simulink model "Controller"  (R2016b)
settings: Solver=ode45  StartTime=0.0  StopTime=330  MaxStep=0.01  RelTol=1e-3  EnableMultiTasking=on
values from neighbouring files (symbols this model uses):
  Controller_d_xc = 25.79    [Variables.m]
  Controller_d_yc = 0    [Variables.m]
  Controller_H = 115    [Variables.m]
  Controller_I_3 = 653.657    [Variables.m]
  Controller_I_L = 351.882    [Variables.m]
  Controller_I_p = 6428.68    [Variables.m]
  Controller_I_R = 351.882    [Variables.m]
  Controller_I_w3 = 628.378    [Variables.m]
  Controller_I_wL = 628.378    [Variables.m]
  Controller_I_wR = 628.378    [Variables.m]
  Controller_L = 107.8    [Variables.m]
  Controller_m_3 = 0.55    [Variables.m]
  Controller_m_L = 1.15    [Variables.m]
  Controller_m_p = 0.75    [Variables.m]
  Controller_m_R = 1.15    [Variables.m]
  Controller_R = 107.8    [Variables.m]
  Controller_R_3 = 50    [Variables.m]
  Controller_R_L = 50    [Variables.m]
  Controller_R_R = 50    [Variables.m]
  d_xc = 25    [Variables.m]
  d_yc = 0    [Variables.m]
  H = 115    [Variables.m]
  I_3 = 655    [Variables.m]
  I_L = 350    [Variables.m]
  I_p = 6430    [Variables.m]
  I_R = 350    [Variables.m]
  I_w3 = 629    [Variables.m]
  I_wL = 629    [Variables.m]
  I_wR = 629    [Variables.m]
  K_eta = diag([1, 1]) * 1.732    [Variables.m]
  K_eta_d = diag([1, 1]) * 0.5    [Variables.m]
  K_eta_i = diag([1, 1]) * 0.5    [Variables.m]
  K_theta = 0.016    [Variables.m]
  K_x = 10    [Variables.m]
  K_y = 0.000064    (= 6.4e-05)    [Variables.m]
  L = 108    [Variables.m]
  m_3 = 0.6    [Variables.m]
  m_L = 1.2    [Variables.m]
  m_p = 0.8    [Variables.m]
  m_R = 1.2    [Variables.m]
  maxTorque = 0    [Variables.m]
  R = 108    [Variables.m]
  R_3 = 52    [Variables.m]
  R_L = 49    [Variables.m]
  R_R = 51    [Variables.m]
undefined symbols (not defined in the file or in its folder): magnitude
settings Model: Creator=Vaibhav Gupta  LastModifiedBy=gupta
settings DataIOCC: ExternalInput=traj  LimitDataPoints=on  LoadExternalInput=on  SaveFormat=Array
settings OptimizationCC: LifeSpan=inf
settings DebuggingCC: SFUnexpectedBacktrackingDiag=warning  SFNoUnconditionalDefaultTransitionDiag=warning  SFExecutionAtInitializationDiag=none
settings HardwareCC: ProdBitPerPointer=32  ProdBitPerSizeT=32  ProdBitPerPtrDiffT=32  ProdLargestAtomicFloat=None  ProdIntDivRoundTo=Undefined  ProdEndianess=Unspecified  ProdWordSize=32  ProdHWDeviceType=32-bit Generic
settings ModelReferenceCC: PropagateSignalLabelsOutOfModel=off
settings GRTTargetCC: TargetLangStandard=C89/C90 (ANSI)  GeneratePreprocessorConditionals=Disable all
settings ConfigComp: CovMetricSettings=dw  CovHtmlReporting=on  CovSaveCumulativeToWorkspaceVar=on  CovSaveSingleToWorkspaceVar=on  CovExternalEMLEnable=off
settings ConfigurationSet: Description=SimMechanics 2G

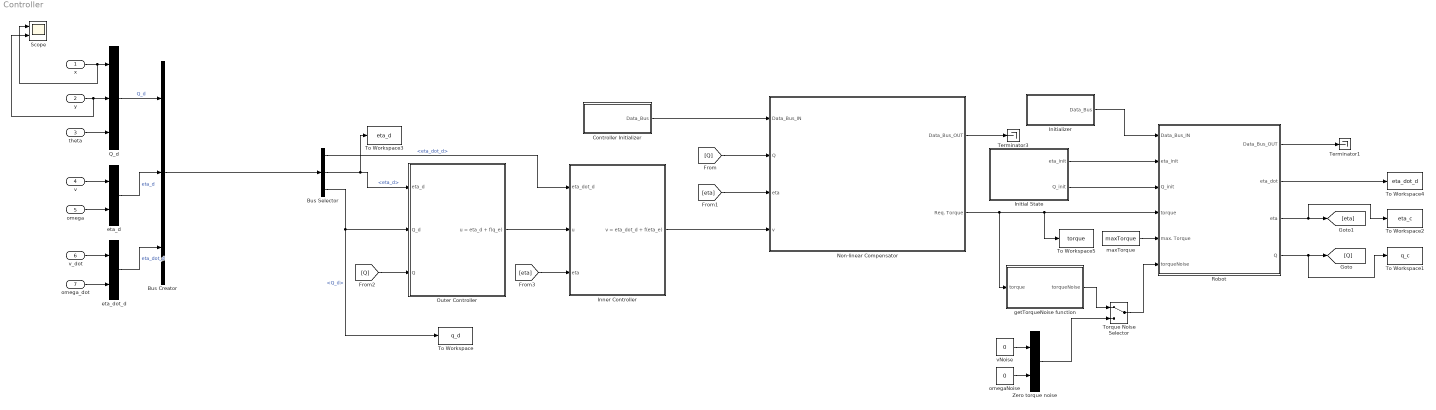
== system Controller ==
  x : Inport
  y : Inport  Port=2
  theta : Inport  Port=3
  v : Inport  Port=4
  omega : Inport  Port=5
  v_dot : Inport  Port=6
  omega_dot : Inport  Port=7
  Bus Creator : BusCreator  Inputs=3
  Bus Selector : BusSelector  OutputSignals=eta_dot_d,eta_d,Q_d
  Controller Initializer : Subsystem
  Initial State : Subsystem
  Initializer : Subsystem
  Inner Controller : Subsystem
  Non-linear Compensator : Subsystem
  Outer Controller : Subsystem
  Q_d : Concatenate  NumInputs=3
  Robot : Subsystem
  Scope : Scope  NumInputPorts=2
  Terminator1 : Terminator
  Terminator3 : Terminator
  To Workspace : ToWorkspace  VariableName=q_d  SaveFormat=Structure With Time  SampleTime=-1
      settings: Decimation=2
  To Workspace1 : ToWorkspace  VariableName=q_c  SaveFormat=Structure With Time  SampleTime=-1
      settings: Decimation=2
  To Workspace2 : ToWorkspace  VariableName=eta_c  SaveFormat=Structure With Time  SampleTime=-1
      settings: Decimation=2
  To Workspace3 : ToWorkspace  VariableName=eta_d  SaveFormat=Structure With Time  SampleTime=-1
      settings: Decimation=2
  To Workspace4 : ToWorkspace  VariableName=eta_dot_d  SaveFormat=Structure With Time  SampleTime=-1
      settings: Decimation=2
  To Workspace5 : ToWorkspace  VariableName=torque  SaveFormat=Structure With Time  SampleTime=-1
      settings: Decimation=2
  Torque Noise Selector : ManualSwitch
  Zero torque noise : Concatenate
  eta_d : Concatenate
  eta_dot_d : Concatenate
  getTorqueNoise function : MATLAB Function  TreatAsAtomicUnit=on
  maxTorque : Constant  Value=maxTorque
  omegaNoise : Constant  Value=0
  vNoise : Constant  Value=0
  wires:
  Robot/4(Q) -> To Workspace1/1, [Q]
  Robot/3(eta) -> [eta], To Workspace2/1
  Robot/1(Data_Bus_OUT) -> Terminator1/1
  Non-linear Compensator/2(Req. Torque) -> getTorqueNoise function/1(torque), To Workspace5/1, Robot/4(torque)
  [eta] -> Inner Controller/3(eta)
  [Q] -> Outer Controller/3(Q)
  Outer Controller/1(u = eta_d + f(q_e)) -> Inner Controller/2(u)
  Controller Initializer/1(Data_Bus) -> Non-linear Compensator/1(Data_Bus_IN)
  [eta] -> Non-linear Compensator/3(eta)
  [Q] -> Non-linear Compensator/2(Q)
  Inner Controller/1(v = eta_dot_d + f(eta_e)) -> Non-linear Compensator/4(v)
  Bus Selector/1 -> Inner Controller/1(eta_dot_d)  "<eta_dot_d>"
  Bus Selector/3 -> To Workspace/1, Outer Controller/2(Q_d)  "<Q_d>"
  Bus Selector/2 -> To Workspace3/1, Outer Controller/1(eta_d)  "<eta_d>"
  Initial State/1(eta_init) -> Robot/2(eta_init)
  Initial State/2(Q_init) -> Robot/3(Q_init)
  Bus Creator/1 -> Bus Selector/1
  Robot/2(eta_dot) -> To Workspace4/1
  v_dot/1 -> eta_dot_d/1
  omega/1 -> eta_d/2
  omega_dot/1 -> eta_dot_d/2
  theta/1 -> Q_d/3
  eta_dot_d/1 -> Bus Creator/3  "eta_dot_d"
  Q_d/1 -> Bus Creator/1  "Q_d"
  v/1 -> eta_d/1
  eta_d/1 -> Bus Creator/2  "eta_d"
  y/1 -> Scope/2, Q_d/2
  x/1 -> Scope/1, Q_d/1
  maxTorque/1 -> Robot/5(max. Torque)
  Initializer/1(Data_Bus) -> Robot/1(Data_Bus_IN)
  Non-linear Compensator/1(Data_Bus_OUT) -> Terminator3/1
  Torque Noise Selector/1 -> Robot/6(torqueNoise)
  getTorqueNoise function/1(torqueNoise) -> Torque Noise Selector/1
  omegaNoise/1 -> Zero torque noise/2
  vNoise/1 -> Zero torque noise/1
  Zero torque noise/1 -> Torque Noise Selector/2

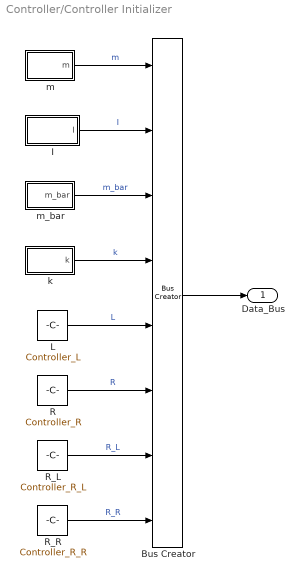
== system Controller/Controller Initializer ==
  Bus Creator : BusCreator  Inputs=8
  I : Subsystem
  L : Constant  Value=Controller_L
  R : Constant  Value=Controller_R
  R_L : Constant  Value=Controller_R_L
  R_R : Constant  Value=Controller_R_R
  k : Subsystem
  m : Subsystem
  m_bar : Subsystem
  Data_Bus : Outport
  wires:
  R_R/1 -> Bus Creator/8  "R_R"
  R_L/1 -> Bus Creator/7  "R_L"
  L/1 -> Bus Creator/5  "L"
  R/1 -> Bus Creator/6  "R"
  k/1(k) -> Bus Creator/4  "k"
  m/1(m) -> Bus Creator/1  "m"
  Bus Creator/1 -> Data_Bus/1
  m_bar/1(m_bar) -> Bus Creator/3  "m_bar"
  I/1(I) -> Bus Creator/2  "I"

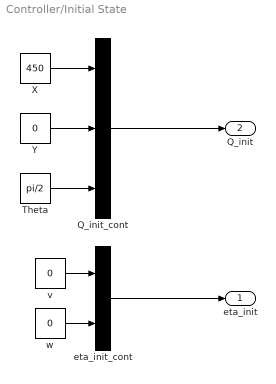
== system Controller/Initial State ==
  Q_init_cont : Concatenate  NumInputs=3
  Theta : Constant  Value=pi/2
  X : Constant  Value=450
  Y : Constant  Value=0
  eta_init_cont : Concatenate
  v : Constant  Value=0
  w : Constant  Value=0
  eta_init : Outport
  Q_init : Outport  Port=2
  wires:
  w/1 -> eta_init_cont/2
  Y/1 -> Q_init_cont/2
  Theta/1 -> Q_init_cont/3
  v/1 -> eta_init_cont/1
  X/1 -> Q_init_cont/1
  Q_init_cont/1 -> Q_init/1
  eta_init_cont/1 -> eta_init/1

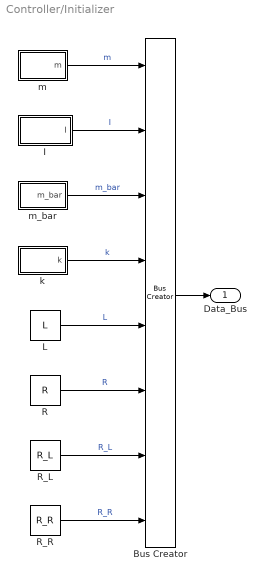
== system Controller/Initializer ==
  Bus Creator : BusCreator  Inputs=8
  I : Subsystem
  L : Constant  Value=L
  R : Constant  Value=R
  R_L : Constant  Value=R_L
  R_R : Constant  Value=R_R
  k : Subsystem
  m : Subsystem
  m_bar : Subsystem
  Data_Bus : Outport
  wires:
  I/1(I) -> Bus Creator/2  "I"
  m_bar/1(m_bar) -> Bus Creator/3  "m_bar"
  Bus Creator/1 -> Data_Bus/1
  m/1(m) -> Bus Creator/1  "m"
  k/1(k) -> Bus Creator/4  "k"
  R/1 -> Bus Creator/6  "R"
  L/1 -> Bus Creator/5  "L"
  R_L/1 -> Bus Creator/7  "R_L"
  R_R/1 -> Bus Creator/8  "R_R"

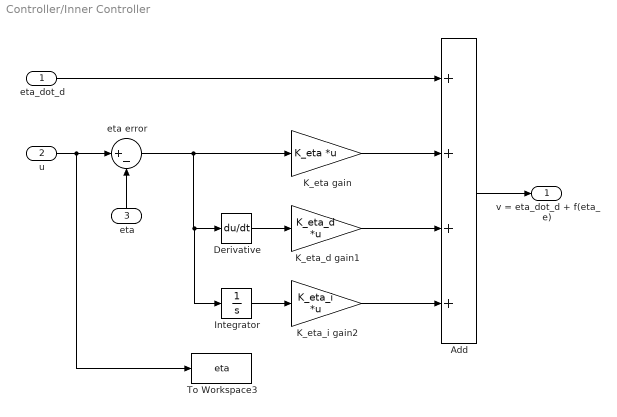
== system Controller/Inner Controller ==
  eta_dot_d : Inport
  u : Inport  Port=2
  eta : Inport  Port=3
  Add : Sum  Inputs=++++
  Derivative : Derivative  CoefficientInTFapproximation=100
  Integrator : Integrator  LimitOutput=on  UpperSaturationLimit=100  LowerSaturationLimit=-100
  K_eta gain : Gain  Gain=K_eta  Multiplication=Matrix(K*u) (u vector)
  K_eta_d gain1 : Gain  Gain=K_eta_d  Multiplication=Matrix(K*u) (u vector)
  K_eta_i gain2 : Gain  Gain=K_eta_i  Multiplication=Matrix(K*u) (u vector)
  To Workspace3 : ToWorkspace  VariableName=eta  SaveFormat=Structure With Time  SampleTime=-1
      settings: Decimation=2
  eta error : Sum  Inputs=|+-
  v = eta_dot_d + f(eta_e) : Outport
  wires:
  Add/1 -> v = eta_dot_d + f(eta_e)/1
  eta_dot_d/1 -> Add/1
  K_eta gain/1 -> Add/2
  eta error/1 -> Integrator/1, Derivative/1, K_eta gain/1
  u/1 -> To Workspace3/1, eta error/1
  eta/1 -> eta error/2
  K_eta_d gain1/1 -> Add/3
  Derivative/1 -> K_eta_d gain1/1
  Integrator/1 -> K_eta_i gain2/1
  K_eta_i gain2/1 -> Add/4

== system Controller/Non-linear Compensator ==
  Data_Bus_IN : Inport
  Q : Inport  Port=2
  eta : Inport  Port=3
  v : Inport  Port=4
  Bus Selector1 : BusSelector  OutputSignals=m,I,m_bar,k,L,R,R_L,R_R
  getTorque function : MATLAB Function  TreatAsAtomicUnit=on
  Data_Bus_OUT : Outport
  Req. Torque : Outport  Port=2
  wires:
  getTorque function/1(torque) -> Req. Torque/1
  Data_Bus_IN/1 -> Bus Selector1/1, Data_Bus_OUT/1
  v/1 -> getTorque function/11(v)
  eta/1 -> getTorque function/10(eta)
  Q/1 -> getTorque function/9(Q)
  Bus Selector1/1 -> getTorque function/1(M)  "<m>"
  Bus Selector1/2 -> getTorque function/2(I)  "<I>"
  Bus Selector1/3 -> getTorque function/3(M_bar)  "<m_bar>"
  Bus Selector1/4 -> getTorque function/4(k)  "<k>"
  Bus Selector1/5 -> getTorque function/5(L)  "<L>"
  Bus Selector1/6 -> getTorque function/6(R)  "<R>"
  Bus Selector1/7 -> getTorque function/7(R_L)  "<R_L>"
  Bus Selector1/8 -> getTorque function/8(R_R)  "<R_R>"

== system Controller/Outer Controller ==
  eta_d : Inport
  Q_d : Inport  Port=2
  Q : Inport  Port=3
  K_theta : Constant  Value=K_theta
  K_x : Constant  Value=K_x
  K_y : Constant  Value=K_y
  Q error : Sum  Inputs=|+-
  getX function : MATLAB Function  TreatAsAtomicUnit=on
  u = eta_d + f(q_e) : Outport
  wires:
  Q_d/1 -> Q error/1
  Q/1 -> getX function/6(Q), Q error/2
  Q error/1 -> getX function/5(Q_e)
  eta_d/1 -> getX function/1(eta_d)
  getX function/1(x) -> u = eta_d + f(q_e)/1
  K_x/1 -> getX function/2(K_x)
  K_y/1 -> getX function/3(K_y)
  K_theta/1 -> getX function/4(K_theta)

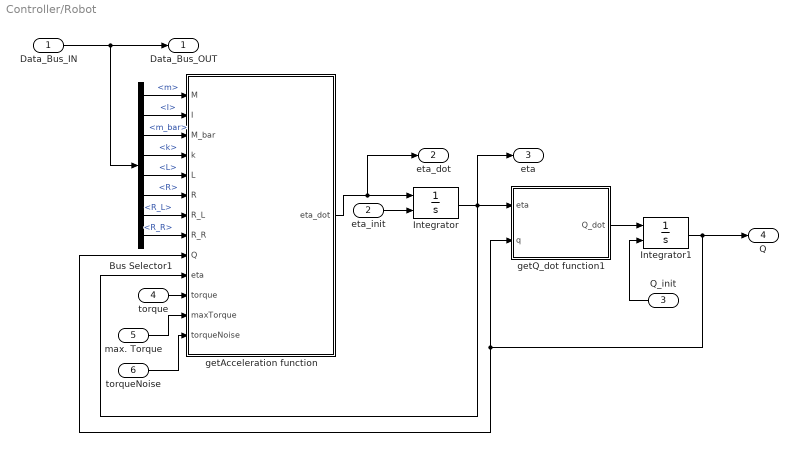
== system Controller/Robot ==
  Data_Bus_IN : Inport
  eta_init : Inport  Port=2
  Q_init : Inport  Port=3
  torque : Inport  Port=4
  max. Torque : Inport  Port=5
  torqueNoise : Inport  Port=6
  Bus Selector1 : BusSelector  OutputSignals=m,I,m_bar,k,L,R,R_L,R_R
  Integrator : Integrator  InitialConditionSource=external  UpperSaturationLimit=10  LowerSaturationLimit=-10
  Integrator1 : Integrator  InitialConditionSource=external
  getAcceleration function : MATLAB Function  TreatAsAtomicUnit=on
  getQ_dot function1 : MATLAB Function  TreatAsAtomicUnit=on
  Data_Bus_OUT : Outport
  eta_dot : Outport  Port=2
  eta : Outport  Port=3
  Q : Outport  Port=4
  wires:
  Integrator/1 -> getQ_dot function1/1(eta), getAcceleration function/10(eta), eta/1
  Integrator1/1 -> getQ_dot function1/2(q), getAcceleration function/9(Q), Q/1
  Bus Selector1/1 -> getAcceleration function/1(M)  "<m>"
  Q_init/1 -> Integrator1/2
  eta_init/1 -> Integrator/2
  torque/1 -> getAcceleration function/11(torque)
  Bus Selector1/2 -> getAcceleration function/2(I)  "<I>"
  Data_Bus_IN/1 -> Bus Selector1/1, Data_Bus_OUT/1
  getAcceleration function/1(eta_dot) -> Integrator/1, eta_dot/1
  Bus Selector1/3 -> getAcceleration function/3(M_bar)  "<m_bar>"
  Bus Selector1/4 -> getAcceleration function/4(k)  "<k>"
  Bus Selector1/5 -> getAcceleration function/5(L)  "<L>"
  Bus Selector1/6 -> getAcceleration function/6(R)  "<R>"
  Bus Selector1/7 -> getAcceleration function/7(R_L)  "<R_L>"
  Bus Selector1/8 -> getAcceleration function/8(R_R)  "<R_R>"
  getQ_dot function1/1(Q_dot) -> Integrator1/1
  max. Torque/1 -> getAcceleration function/12(maxTorque)
  torqueNoise/1 -> getAcceleration function/13(torqueNoise)

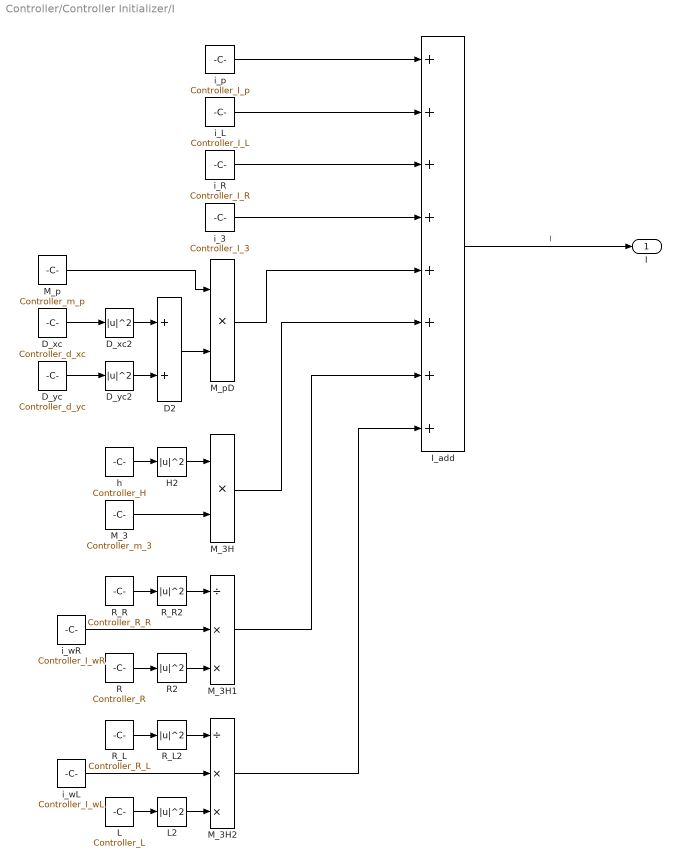
== system Controller/Controller Initializer/I ==
  D2 : Sum
  D_xc : Constant  Value=Controller_d_xc
  D_xc2 : Math  Operator=magnitude^2  SaturateOnIntegerOverflow=on
  D_yc : Constant  Value=Controller_d_yc
  D_yc2 : Math  Operator=magnitude^2  SaturateOnIntegerOverflow=on
  H2 : Math  Operator=magnitude^2  SaturateOnIntegerOverflow=on
  I_add : Sum  Inputs=++++++++
  L : Constant  Value=Controller_L
  L2 : Math  Operator=magnitude^2  SaturateOnIntegerOverflow=on
  M_3 : Constant  Value=Controller_m_3
  M_3H : Product  Inputs=**
  M_3H1 : Product  Inputs=/**
  M_3H2 : Product  Inputs=/**
  M_p : Constant  Value=Controller_m_p
  M_pD : Product  Inputs=**
  R : Constant  Value=Controller_R
  R2 : Math  Operator=magnitude^2  SaturateOnIntegerOverflow=on
  R_L : Constant  Value=Controller_R_L
  R_L2 : Math  Operator=magnitude^2  SaturateOnIntegerOverflow=on
  R_R : Constant  Value=Controller_R_R
  R_R2 : Math  Operator=magnitude^2  SaturateOnIntegerOverflow=on
  h : Constant  Value=Controller_H
  i_3 : Constant  Value=Controller_I_3
  i_L : Constant  Value=Controller_I_L
  i_R : Constant  Value=Controller_I_R
  i_p : Constant  Value=Controller_I_p
  i_wL : Constant  Value=Controller_I_wL
  i_wR : Constant  Value=Controller_I_wR
  I : Outport
  wires:
  i_wL/1 -> M_3H2/2
  L2/1 -> M_3H2/3
  L/1 -> L2/1
  R_L2/1 -> M_3H2/1
  R_L/1 -> R_L2/1
  M_3H2/1 -> I_add/8
  i_wR/1 -> M_3H1/2
  R2/1 -> M_3H1/3
  R/1 -> R2/1
  R_R2/1 -> M_3H1/1
  R_R/1 -> R_R2/1
  M_3H1/1 -> I_add/7
  i_p/1 -> I_add/1
  i_L/1 -> I_add/2
  i_R/1 -> I_add/3
  i_3/1 -> I_add/4
  I_add/1 -> I/1  "I"
  M_p/1 -> M_pD/1
  D_xc/1 -> D_xc2/1
  D_yc/1 -> D_yc2/1
  D_xc2/1 -> D2/1
  D_yc2/1 -> D2/2
  D2/1 -> M_pD/2
  M_pD/1 -> I_add/5
  H2/1 -> M_3H/1
  h/1 -> H2/1
  M_3/1 -> M_3H/2
  M_3H/1 -> I_add/6

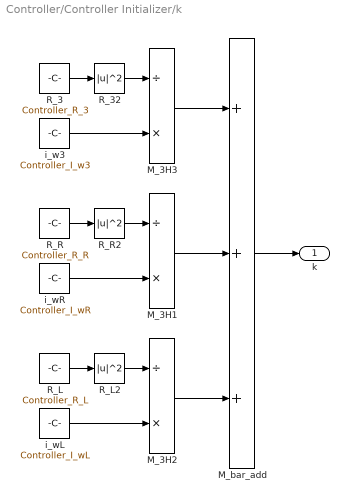
== system Controller/Controller Initializer/k ==
  M_3H1 : Product  Inputs=/*
  M_3H2 : Product  Inputs=/*
  M_3H3 : Product  Inputs=/*
  M_bar_add : Sum  Inputs=+++
  R_3 : Constant  Value=Controller_R_3
  R_32 : Math  Operator=magnitude^2  SaturateOnIntegerOverflow=on
  R_L : Constant  Value=Controller_R_L
  R_L2 : Math  Operator=magnitude^2  SaturateOnIntegerOverflow=on
  R_R : Constant  Value=Controller_R_R
  R_R2 : Math  Operator=magnitude^2  SaturateOnIntegerOverflow=on
  i_w3 : Constant  Value=Controller_I_w3
  i_wL : Constant  Value=Controller_I_wL
  i_wR : Constant  Value=Controller_I_wR
  k : Outport
  wires:
  M_3H3/1 -> M_bar_add/1
  i_w3/1 -> M_3H3/2
  R_32/1 -> M_3H3/1
  R_3/1 -> R_32/1
  M_3H1/1 -> M_bar_add/2
  M_3H2/1 -> M_bar_add/3
  i_wL/1 -> M_3H2/2
  R_L2/1 -> M_3H2/1
  R_L/1 -> R_L2/1
  i_wR/1 -> M_3H1/2
  R_R2/1 -> M_3H1/1
  R_R/1 -> R_R2/1
  M_bar_add/1 -> k/1

== system Controller/Controller Initializer/m ==
  M_3 : Constant  Value=Controller_m_3
  M_L : Constant  Value=Controller_m_L
  M_R : Constant  Value=Controller_m_R
  M_add : Sum  Inputs=++++
  M_p : Constant  Value=Controller_m_p
  m : Outport
  wires:
  M_3/1 -> M_add/4
  M_L/1 -> M_add/2
  M_p/1 -> M_add/1
  M_R/1 -> M_add/3
  M_add/1 -> m/1  "m"

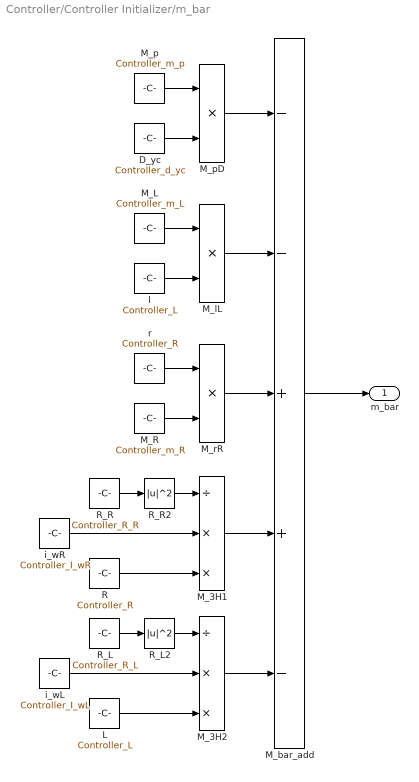
== system Controller/Controller Initializer/m_bar ==
  D_yc : Constant  Value=Controller_d_yc
  L : Constant  Value=Controller_L
  M_3H1 : Product  Inputs=/**
  M_3H2 : Product  Inputs=/**
  M_L : Constant  Value=Controller_m_L
  M_R : Constant  Value=Controller_m_R
  M_bar_add : Sum  Inputs=--++-
  M_lL : Product  Inputs=**
  M_p : Constant  Value=Controller_m_p
  M_pD : Product  Inputs=**
  M_rR : Product  Inputs=**
  R : Constant  Value=Controller_R
  R_L : Constant  Value=Controller_R_L
  R_L2 : Math  Operator=magnitude^2  SaturateOnIntegerOverflow=on
  R_R : Constant  Value=Controller_R_R
  R_R2 : Math  Operator=magnitude^2  SaturateOnIntegerOverflow=on
  i_wL : Constant  Value=Controller_I_wL
  i_wR : Constant  Value=Controller_I_wR
  l : Constant  Value=Controller_L
  r : Constant  Value=Controller_R
  m_bar : Outport
  wires:
  M_3H1/1 -> M_bar_add/4
  M_3H2/1 -> M_bar_add/5
  i_wL/1 -> M_3H2/2
  L/1 -> M_3H2/3
  R_L2/1 -> M_3H2/1
  R_L/1 -> R_L2/1
  i_wR/1 -> M_3H1/2
  R/1 -> M_3H1/3
  R_R2/1 -> M_3H1/1
  R_R/1 -> R_R2/1
  D_yc/1 -> M_pD/2
  M_p/1 -> M_pD/1
  l/1 -> M_lL/2
  M_L/1 -> M_lL/1
  M_R/1 -> M_rR/2
  r/1 -> M_rR/1
  M_pD/1 -> M_bar_add/1
  M_lL/1 -> M_bar_add/2
  M_rR/1 -> M_bar_add/3
  M_bar_add/1 -> m_bar/1

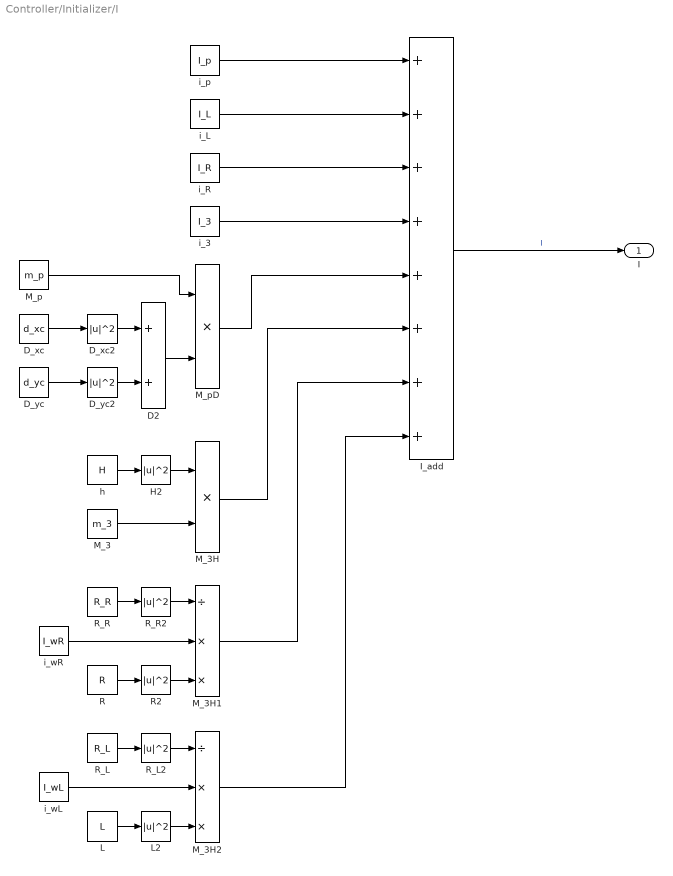
== system Controller/Initializer/I ==
  D2 : Sum
  D_xc : Constant  Value=d_xc
  D_xc2 : Math  Operator=magnitude^2  SaturateOnIntegerOverflow=on
  D_yc : Constant  Value=d_yc
  D_yc2 : Math  Operator=magnitude^2  SaturateOnIntegerOverflow=on
  H2 : Math  Operator=magnitude^2  SaturateOnIntegerOverflow=on
  I_add : Sum  Inputs=++++++++
  L : Constant  Value=L
  L2 : Math  Operator=magnitude^2  SaturateOnIntegerOverflow=on
  M_3 : Constant  Value=m_3
  M_3H : Product  Inputs=**
  M_3H1 : Product  Inputs=/**
  M_3H2 : Product  Inputs=/**
  M_p : Constant  Value=m_p
  M_pD : Product  Inputs=**
  R : Constant  Value=R
  R2 : Math  Operator=magnitude^2  SaturateOnIntegerOverflow=on
  R_L : Constant  Value=R_L
  R_L2 : Math  Operator=magnitude^2  SaturateOnIntegerOverflow=on
  R_R : Constant  Value=R_R
  R_R2 : Math  Operator=magnitude^2  SaturateOnIntegerOverflow=on
  h : Constant  Value=H
  i_3 : Constant  Value=I_3
  i_L : Constant  Value=I_L
  i_R : Constant  Value=I_R
  i_p : Constant  Value=I_p
  i_wL : Constant  Value=I_wL
  i_wR : Constant  Value=I_wR
  I : Outport
  wires:
  M_3H/1 -> I_add/6
  M_3/1 -> M_3H/2
  h/1 -> H2/1
  H2/1 -> M_3H/1
  M_pD/1 -> I_add/5
  D2/1 -> M_pD/2
  D_yc2/1 -> D2/2
  D_xc2/1 -> D2/1
  D_yc/1 -> D_yc2/1
  D_xc/1 -> D_xc2/1
  M_p/1 -> M_pD/1
  I_add/1 -> I/1  "I"
  i_3/1 -> I_add/4
  i_R/1 -> I_add/3
  i_L/1 -> I_add/2
  i_p/1 -> I_add/1
  M_3H1/1 -> I_add/7
  R_R/1 -> R_R2/1
  R_R2/1 -> M_3H1/1
  R/1 -> R2/1
  R2/1 -> M_3H1/3
  i_wR/1 -> M_3H1/2
  M_3H2/1 -> I_add/8
  R_L/1 -> R_L2/1
  R_L2/1 -> M_3H2/1
  L/1 -> L2/1
  L2/1 -> M_3H2/3
  i_wL/1 -> M_3H2/2

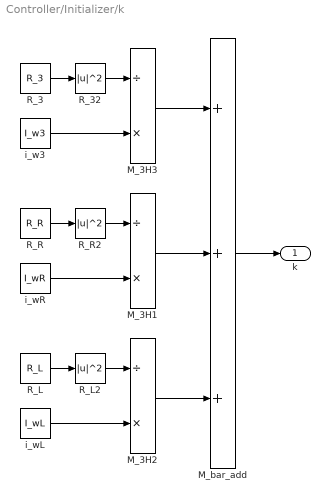
== system Controller/Initializer/k ==
  M_3H1 : Product  Inputs=/*
  M_3H2 : Product  Inputs=/*
  M_3H3 : Product  Inputs=/*
  M_bar_add : Sum  Inputs=+++
  R_3 : Constant  Value=R_3
  R_32 : Math  Operator=magnitude^2  SaturateOnIntegerOverflow=on
  R_L : Constant  Value=R_L
  R_L2 : Math  Operator=magnitude^2  SaturateOnIntegerOverflow=on
  R_R : Constant  Value=R_R
  R_R2 : Math  Operator=magnitude^2  SaturateOnIntegerOverflow=on
  i_w3 : Constant  Value=I_w3
  i_wL : Constant  Value=I_wL
  i_wR : Constant  Value=I_wR
  k : Outport
  wires:
  M_bar_add/1 -> k/1
  R_R/1 -> R_R2/1
  R_R2/1 -> M_3H1/1
  i_wR/1 -> M_3H1/2
  R_L/1 -> R_L2/1
  R_L2/1 -> M_3H2/1
  i_wL/1 -> M_3H2/2
  M_3H2/1 -> M_bar_add/3
  M_3H1/1 -> M_bar_add/2
  R_3/1 -> R_32/1
  R_32/1 -> M_3H3/1
  i_w3/1 -> M_3H3/2
  M_3H3/1 -> M_bar_add/1

== system Controller/Initializer/m ==
  M_3 : Constant  Value=m_3
  M_L : Constant  Value=m_L
  M_R : Constant  Value=m_R
  M_add : Sum  Inputs=++++
  M_p : Constant  Value=m_p
  m : Outport
  wires:
  M_add/1 -> m/1  "m"
  M_R/1 -> M_add/3
  M_p/1 -> M_add/1
  M_L/1 -> M_add/2
  M_3/1 -> M_add/4

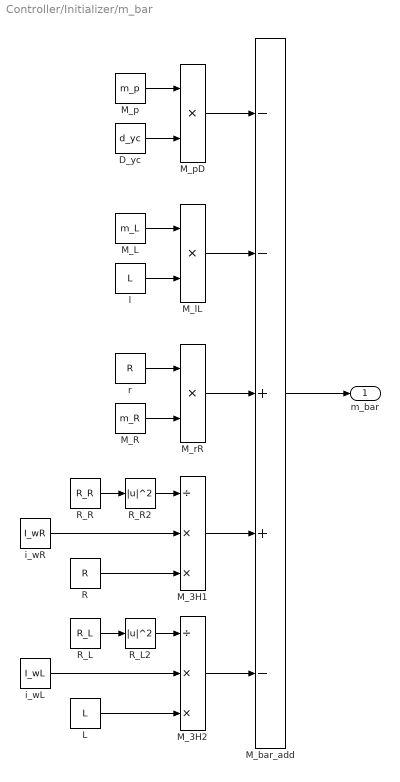
== system Controller/Initializer/m_bar ==
  D_yc : Constant  Value=d_yc
  L : Constant  Value=L
  M_3H1 : Product  Inputs=/**
  M_3H2 : Product  Inputs=/**
  M_L : Constant  Value=m_L
  M_R : Constant  Value=m_R
  M_bar_add : Sum  Inputs=--++-
  M_lL : Product  Inputs=**
  M_p : Constant  Value=m_p
  M_pD : Product  Inputs=**
  M_rR : Product  Inputs=**
  R : Constant  Value=R
  R_L : Constant  Value=R_L
  R_L2 : Math  Operator=magnitude^2  SaturateOnIntegerOverflow=on
  R_R : Constant  Value=R_R
  R_R2 : Math  Operator=magnitude^2  SaturateOnIntegerOverflow=on
  i_wL : Constant  Value=I_wL
  i_wR : Constant  Value=I_wR
  l : Constant  Value=L
  r : Constant  Value=R
  m_bar : Outport
  wires:
  M_bar_add/1 -> m_bar/1
  M_rR/1 -> M_bar_add/3
  M_lL/1 -> M_bar_add/2
  M_pD/1 -> M_bar_add/1
  r/1 -> M_rR/1
  M_R/1 -> M_rR/2
  M_L/1 -> M_lL/1
  l/1 -> M_lL/2
  M_p/1 -> M_pD/1
  D_yc/1 -> M_pD/2
  R_R/1 -> R_R2/1
  R_R2/1 -> M_3H1/1
  R/1 -> M_3H1/3
  i_wR/1 -> M_3H1/2
  R_L/1 -> R_L2/1
  R_L2/1 -> M_3H2/1
  L/1 -> M_3H2/3
  i_wL/1 -> M_3H2/2
  M_3H2/1 -> M_bar_add/5
  M_3H1/1 -> M_bar_add/4

== matlab function Controller/Non-linear Compensator/getTorque function ==
  data: M input; I input; M_bar input; k input; L input; R input; R_L input; R_R input; Q input; eta input; v input; torque output
function torque   = getTorque(M, I, M_bar, k, L, R, R_L, R_R, Q, eta, v)
%% getTorque
% This gives the required value of torque for the motion

theta = Q(3);
sTheta = sin(theta);
cTheta = cos(theta);
dTheta = eta(2);
csTheta = cTheta * sTheta;

M_matrix = [...
    M + k * cTheta^2   , k * csTheta       , M_bar * cTheta     ;
    k * csTheta        , M + k * sTheta^2  , M_bar * sTheta     ;
    M_bar * cTheta     , M_bar * sTheta    , I                  ];


V_matrix = [...
    -k*dTheta*csTheta , -k*dTheta*sTheta^2  , - M_bar*dTheta*sTheta  ;
    k*dTheta*cTheta^2 , k*dTheta*csTheta    , M_bar*dTheta*cTheta    ;
    - dTheta * sTheta , dTheta * cTheta     , 0                      ];
    
B_matrix = [...
    cTheta/R_L	, cTheta/R_R    ;
    sTheta/R_L  , sTheta/R_R    ;
    - L / R_L   , R / R_R       ];

A_matrix = [...
    - sTheta    , cTheta    , 0     ];

S = [...
    cTheta  , 0         ;
    sTheta  , 0         ;
    0       , 1         ];

S_dot = [...
    -sTheta * dTheta    , 0 ;
    cTheta * dTheta     , 0 ;
    0                   , 0 ];

RHS_matrix = [S' * B_matrix];

LHS = S' * M_matrix * S * v + S' * M_matrix * S_dot * eta + S' * V_matrix * S * eta;

RHS_variables =  RHS_matrix \ LHS;
    
torque = RHS_variables;

== matlab function Controller/Robot/getAcceleration function ==
  data: M input; I input; M_bar input; k input; L input; R input; R_L input; R_R input; Q input; eta input; torque input; eta_dot output; maxTorque input; torqueNoise input
function eta_dot  = getAcceleration(M, I, M_bar, k, L, R, R_L, R_R, Q, eta, torque, maxTorque, torqueNoise)
%% getTorque
% This gives the required value of torque for the motion

if (maxTorque ~= 0)
    torque(abs(torque) > maxTorque) = sign(torque(abs(torque) > maxTorque)) * maxTorque;
end

torque = torque + torqueNoise;

theta = Q(3);
sTheta = sin(theta);
cTheta = cos(theta);
dTheta = eta(2);
csTheta = cTheta * sTheta;

M_matrix = [...
    M + k * cTheta^2   , k * csTheta       , M_bar * cTheta     ;
    k * csTheta        , M + k * sTheta^2  , M_bar * sTheta     ;
    M_bar * cTheta     , M_bar * sTheta    , I                  ];

V_matrix = [...
    -k*dTheta*csTheta , -k*dTheta*sTheta^2  , - M_bar*dTheta*sTheta  ;
    k*dTheta*cTheta^2 , k*dTheta*csTheta    , M_bar*dTheta*cTheta    ;
    - dTheta * sTheta , dTheta * cTheta     , 0                      ];
    
B_matrix = [...
    cTheta/R_L	, cTheta/R_R    ;
    sTheta/R_L  , sTheta/R_R    ;
    - L / R_L   , R / R_R       ];

A_matrix = [...
    - sTheta    , cTheta    , 0     ];

S = [...
    cTheta  , 0         ;
    sTheta  , 0         ;
    0       , 1         ];

S_dot = [...
    -sTheta * dTheta    , 0 ;
    cTheta * dTheta     , 0 ;
    0                   , 0 ];

LHS_matrix = [S' * M_matrix * S];

RHS = S' * B_matrix * torque - S' * V_matrix * S * eta - S' * M_matrix * S_dot * eta;

RHS_variables =  LHS_matrix \ RHS;

eta_dot = RHS_variables;

== matlab function Controller/Outer Controller/getX function ==
  data: eta_d input; K_x input; K_y input; K_theta input; Q_e input; x output; Q input
function x   = getX(eta_d, K_x, K_y, K_theta, Q_e, Q)
%% getEta
% return poseError corrections

Theta = Q(3);
q_e = [...
    cos(Theta)  ,   sin(Theta)  ,   0   ;
    -sin(Theta) ,   cos(Theta)  ,   0   ;
    0           ,   0           ,   1   ] * Q_e;

x = [...
    eta_d(1) * cos(q_e(3)) + K_x * q_e(1)                           ;
    eta_d(2) + eta_d(1) * ( K_y * q_e(2) + K_theta * sin(q_e(3)))   ];

== matlab function Controller/Robot/getQ_dot function1 ==
  data: eta input; q input; Q_dot output
function Q_dot  = getQ_dot(eta, q)
%% getTorque
% This gives the required value of torque for the motion

theta = q(3);
sTheta = sin(theta);
cTheta = cos(theta);

S = [...
    cTheta  , 0         ;
    sTheta  , 0         ;
    0       , 1         ];

Q_dot = S * eta;

== matlab function Controller/getTorqueNoise function ==
  data: torque input; torqueNoise output
function torqueNoise = getTorqueNoise(torque)

v_prob = rand * 2 - 1;
omega_prob = rand * 2 - 1;

if (v_prob > 0.75)
    v_prob = 1;
elseif (v_prob < -0.75)
    v_prob = -1;
else
    v_prob = 0;
end

if (omega_prob > 0.75)
    omega_prob = 1;
elseif (omega_prob < -0.75)
    omega_prob = -1;
else
    omega_prob = 0;
end

vNoise = random('norm', 0.01 * torque(1), 1);
omegaNoise = random('norm', 0.01 * torque(2), 1);

torqueNoise = [...
    vNoise * v_prob         ;
    omegaNoise * omega_prob];
end
